simulink model "Servo_PID"  (R2013b)
settings: Solver=ode5  SolverMode=SingleTasking  StartTime=0.0  StopTime=30  FixedStep=0.002  RelTol=1e-3  AbsTol=1e-6
undefined symbols (not defined in the file): a, b, ksi, ksie, lambda, omega, omegae, RTDAC4PCIBaseAddress, Tfiltra, Tsampling
settings Model: SimulationMode=external  ExtModeTrigDuration=20000  ExtModeTrigLevel=0.400000  Creator=jims  LastModifiedBy=Admin
settings DataIOCC: ExternalInput=[]  InitialState=[]  LimitDataPoints=off  MaxDataPoints=5000  SignalLoggingSaveFormat=ModelDataLogs  SaveOutput=off  SaveTime=off  SignalLoggingName=sigsOut
settings OptimizationCC: BooleanDataType=off  ExpressionDepthLimit=2147483647  InitFltsAndDblsToZero=on
settings DebuggingCC: SaveWithParameterizedLinksMsg=none  SignalResolutionControl=TryResolveAllWithWarning  SolverPrmCheckMsg=none  MultiTaskDSMMsg=warning  MultiTaskCondExecSysMsg=none  IntegerOverflowMsg=none  FcnCallInpInsideContextMsg=UseLocalSettings  StateNameClashWarn=warning
settings HardwareCC: ProdIntDivRoundTo=Zero  ProdEndianess=LittleEndian  ProdHWDeviceType=Generic->32-bit x86 compatible
settings RTWCC: SystemTargetFile=rtwin.tlc  TemplateMakefile=rtwin.tmf  Description=Real-Time Windows Target  ProcessScript=rtwin_make_rtw_hook  IncludeERTFirstTime=on  RTWCompilerOptimization=On
settings CodeAppCC: MaxIdLength=95
settings RTWinTargetCC: TargetLibSuffix=_rtwin.lib  TargetPreCompLibLocation=C:\Program Files\MATLAB\R2013b\toolbox\rtw\targets\rtwin\lib\win64  CodeReplacementLibrary=ANSI_C  RTWinDir=C:/PROGRA~1/MATLAB/R2013b/toolbox/rtw/targets/rtwin  TargetArch=win64

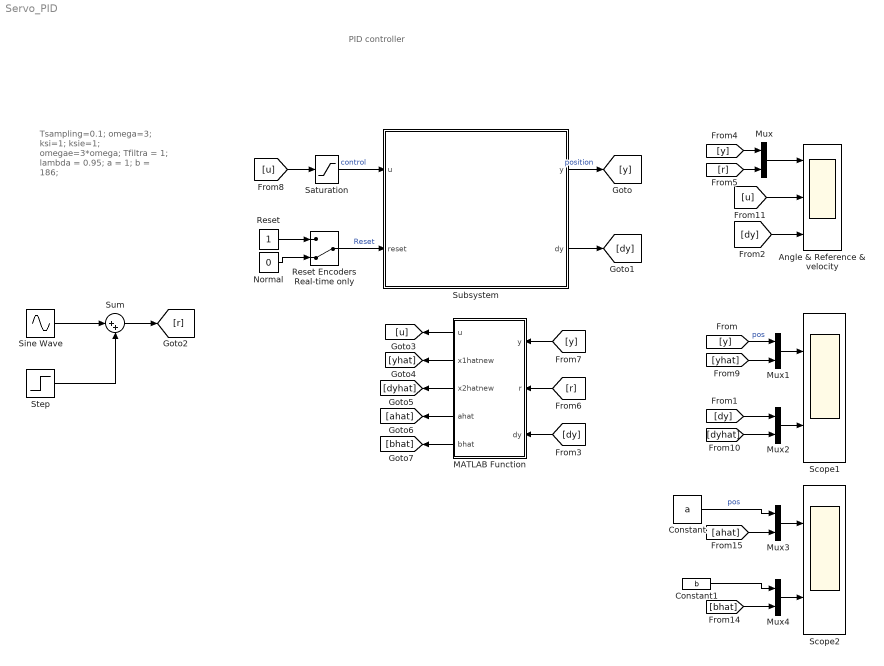
== system Servo_PID ==
  note: Tsampling=0.1;
      | omega=3;
      | ksi=1;
      | ksie=1;
      | omegae=3*omega;
      | Tfiltra = 1;
      | lambda = 0.95;
      | a = 1;
      | b = 186;
  note: PID controller
  Angle & Reference & velocity : Scope  NumInputPorts=3
      settings: ShowLegends=on  TimeRange=30  YMin=250~-0.175~-16  YMax=350~0.075~7  SaveName=PD_C  MaxDataPoints=20000  Decimation=10
  Constant : Constant  Value=a
  Constant1 : Constant  Value=b
  MATLAB Function : MATLAB Function  TreatAsAtomicUnit=on
  Mux{,1..4} (5 alike) : Mux  Inputs=2
  Normal : Constant  Value=0
  Reset : Constant
  Reset Encoders Real-time only : ManualSwitch  CurrentSetting=0
  Saturation : Saturate  UpperLimit=1  LowerLimit=-1
  Scope1 : Scope  NumInputPorts=2
      settings: ShowLegends=on  YMin=275~0  YMax=350~19
  Scope2 : Scope  NumInputPorts=2
      settings: ShowLegends=on  YMin=275~0  YMax=350~19
  Sine Wave : Sin  Amplitude=50  Frequency=2*pi/20  SampleTime=0
  Step : Step  After=300  SampleTime=0
  Subsystem : Subsystem
  Sum : Sum  Inputs=|++
  wires:
  Normal/1 -> Reset Encoders Real-time only/2
  Reset/1 -> Reset Encoders Real-time only/1
  Saturation/1 -> Subsystem/1(u)  "control"
  Reset Encoders Real-time only/1 -> Subsystem/2(reset)  "Reset"
  Mux/1 -> Angle & Reference & velocity/1
  Subsystem/2(dy) -> [dy]
  Subsystem/1(y) -> [y]  "position"
  [dy] -> Angle & Reference & velocity/3
  [dy] -> MATLAB Function/3(dy)
  [y] -> Mux/1
  Sine Wave/1 -> Sum/1
  Step/1 -> Sum/2
  Sum/1 -> [r]
  [r] -> Mux/2
  [r] -> MATLAB Function/2(r)
  [y] -> MATLAB Function/1(y)
  MATLAB Function/1(u) -> [u]
  [u] -> Saturation/1
  Mux1/1 -> Scope1/1
  Mux2/1 -> Scope1/2
  [y] -> Mux1/1  "pos"
  [dy] -> Mux2/1
  MATLAB Function/2(x1hatnew) -> [yhat]
  MATLAB Function/3(x2hatnew) -> [dyhat]
  [yhat] -> Mux1/2
  [dyhat] -> Mux2/2
  [u] -> Angle & Reference & velocity/2
  MATLAB Function/4(ahat) -> [ahat]
  MATLAB Function/5(bhat) -> [bhat]
  Mux3/1 -> Scope2/1
  Mux4/1 -> Scope2/2
  Constant/1 -> Mux3/1  "pos"
  Constant1/1 -> Mux4/1
  [ahat] -> Mux3/2
  [bhat] -> Mux4/2

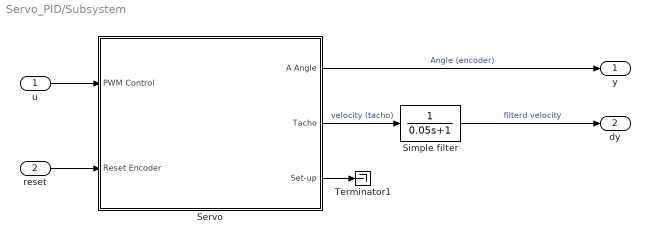
== system Servo_PID/Subsystem ==
  u : Inport
  reset : Inport  Port=2
  Servo : Subsystem  mask{BaseAddress=RTDAC4PCIBaseAddress(-1,-1), T0=0.002}
      mask prompts: BaseAddress "Base Address:"; T0 "Sampling Period:"
      mask Display: image(imread('Servo.JPG'))
  Simple filter : TransferFcn  Denominator=[0.05 1]
  Terminator1 : Terminator
  y : Outport
  dy : Outport  Port=2
  wires:
  Simple filter/1 -> dy/1  "filterd velocity"
  Servo/1(A Angle) -> y/1  "Angle (encoder)"
  reset/1 -> Servo/2(Reset Encoder)
  Servo/2(Tacho) -> Simple filter/1  "velocity (tacho)"
  Servo/3(Set-up) -> Terminator1/1
  u/1 -> Servo/1(PWM Control)

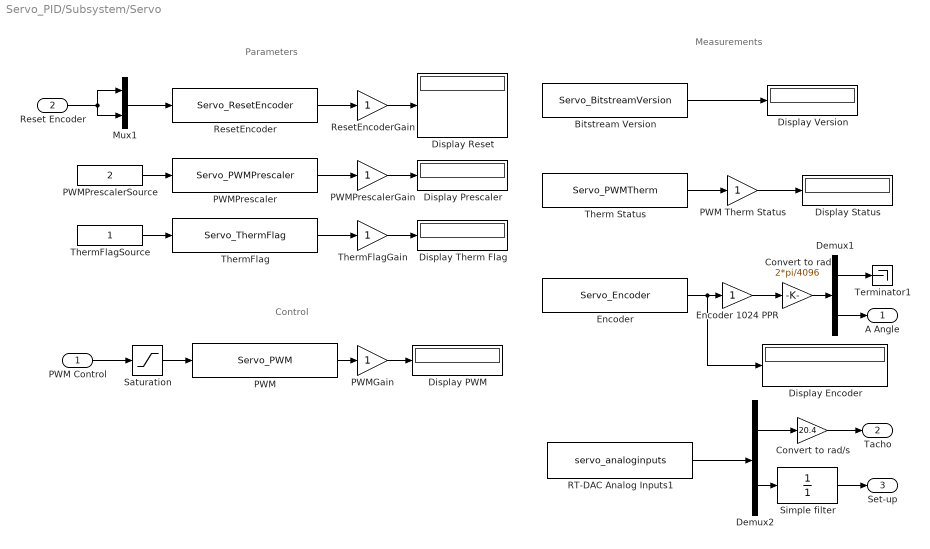
== system Servo_PID/Subsystem/Servo ==
  note: Parameters
  note: Control
  note: Measurements
  PWM Control : Inport
  Reset Encoder : Inport  Port=2
  Bitstream Version : S-Function  FunctionName=Servo_BitstreamVersion  Parameters=BaseAddress, T0  EnableBusSupport=off
  Convert to rad : Gain  Gain=2*pi/4096  SaturateOnIntegerOverflow=on  OutDataTypeStr=Inherit: Same as input  ParamDataTypeStr=Inherit: Same as input
  Convert to rad/s : Gain  Gain=20.4  SaturateOnIntegerOverflow=on  OutDataTypeStr=Inherit: Same as input  ParamDataTypeStr=Inherit: Same as input
  Demux1 : Demux  Outputs=2
  Demux2 : Demux  Outputs=2
  Display Encoder : Display
  Display PWM : Display
  Display Prescaler : Display
  Display Reset : Display
  Display Status : Display
  Display Therm Flag : Display
  Display Version : Display
  Encoder : S-Function  FunctionName=Servo_Encoder  Parameters=BaseAddress, T0  EnableBusSupport=off
  Encoder 1024 PPR : Gain  SaturateOnIntegerOverflow=on  OutDataTypeStr=Inherit: Same as input  ParamDataTypeStr=Inherit: Same as input
  Mux1 : Mux  Inputs=2
  PWM : S-Function  FunctionName=Servo_PWM  Parameters=BaseAddress, T0  EnableBusSupport=off
  PWM Therm Status : Gain  SaturateOnIntegerOverflow=on  OutDataTypeStr=Inherit: Same as input  ParamDataTypeStr=Inherit: Same as input
  PWMGain : Gain  SaturateOnIntegerOverflow=on  OutDataTypeStr=Inherit: Same as input  ParamDataTypeStr=Inherit: Same as input
  PWMPrescaler : S-Function  FunctionName=Servo_PWMPrescaler  Parameters=BaseAddress, T0  EnableBusSupport=off
  PWMPrescalerGain : Gain  SaturateOnIntegerOverflow=on  OutDataTypeStr=Inherit: Same as input  ParamDataTypeStr=Inherit: Same as input
  PWMPrescalerSource : Constant  Value=2
  RT-DAC Analog Inputs1 : S-Function  FunctionName=servo_analoginputs  Parameters=BaseAddress, [1 0], [1 1], T0  EnableBusSupport=off
  ResetEncoder : S-Function  FunctionName=Servo_ResetEncoder  Parameters=BaseAddress, T0  EnableBusSupport=off
  ResetEncoderGain : Gain  SaturateOnIntegerOverflow=on  OutDataTypeStr=Inherit: Same as input  ParamDataTypeStr=Inherit: Same as input
  Saturation : Saturate  UpperLimit=1  LowerLimit=-1
  Simple filter : TransferFcn  Denominator=[0.0 1]
  Terminator1 : Terminator
  Therm Status : S-Function  FunctionName=Servo_PWMTherm  Parameters=BaseAddress, T0  EnableBusSupport=off
  "ThermFlag " : S-Function  FunctionName=Servo_ThermFlag  Parameters=BaseAddress, T0  EnableBusSupport=off
  ThermFlagGain : Gain  SaturateOnIntegerOverflow=on  OutDataTypeStr=Inherit: Same as input  ParamDataTypeStr=Inherit: Same as input
  ThermFlagSource : Constant
  A Angle : Outport
  Tacho : Outport  Port=2
  Set-up : Outport  Port=3
  wires:
  Encoder 1024 PPR/1 -> Convert to rad/1
  Encoder/1 -> Encoder 1024 PPR/1, Display Encoder/1
  Saturation/1 -> PWM/1
  PWM/1 -> PWMGain/1
  PWMGain/1 -> Display PWM/1
  ResetEncoder/1 -> ResetEncoderGain/1
  PWMPrescaler/1 -> PWMPrescalerGain/1
  Mux1/1 -> ResetEncoder/1
  PWMPrescalerSource/1 -> PWMPrescaler/1
  ResetEncoderGain/1 -> Display Reset/1
  PWMPrescalerGain/1 -> Display Prescaler/1
  PWM Control/1 -> Saturation/1
  Convert to rad/1 -> Demux1/1
  Therm Status/1 -> PWM Therm Status/1
  PWM Therm Status/1 -> Display Status/1
  Bitstream Version/1 -> Display Version/1
  Reset Encoder/1 -> Mux1/1, Mux1/2
  "ThermFlag "/1 -> ThermFlagGain/1
  ThermFlagSource/1 -> "ThermFlag "/1
  ThermFlagGain/1 -> Display Therm Flag/1
  Demux1/1 -> Terminator1/1
  Demux1/2 -> A Angle/1
  RT-DAC Analog Inputs1/1 -> Demux2/1
  Demux2/2 -> Simple filter/1
  Demux2/1 -> Convert to rad/s/1
  Convert to rad/s/1 -> Tacho/1
  Simple filter/1 -> Set-up/1

== matlab function Servo_PID/MATLAB Function ==
  settings: updateMethod=DISCRETE  sampleTime=Tsampling
  data: u output; y input; r input; Tsampling parameter; omega parameter; ksi parameter; dy input; omegae parameter; ksie parameter; x1hatnew output; x2hatnew output; Tfiltra parameter; lambda parameter; ahat output; bhat output
function [u, x1hatnew, x2hatnew, ahat, bhat] = fcn(y, r, Tsampling, omega, ksi, dy, omegae, ksie, Tfiltra, lambda)

persistent x1hat x2hat uprev
if isempty(x1hat) || isempty(x2hat) || isempty(uprev)
    x1hat=0;
    x2hat=0;
    uprev = 0;
end

persistent ufp x2fp
if isempty(ufp)
    ufp = 0;
    x2fp = 0;
end

% Filtering
p = exp(-Tsampling/Tfiltra);

uf = p * ufp + (1-p) * uprev;
ufp = uf;

x2f = p * x2fp + (1-p) * dy;
dx2f = (x2f - x2fp)/Tsampling;
x2fp = x2f;

% Kalman
persistent P theta
if isempty(P)
    P = 50*eye(2);
    theta = [0 0]';
end

phi = [-x2f uf]';
z = dx2f;
P = (1/lambda) * (P + (P'*(phi*phi')*P)/(lambda + phi'*P*phi));
theta = theta + P*phi*(z-phi'*theta);
ahat = theta(1);
bhat = theta(2);


% Control & observer
a=1;
b=186;

k1=omega^2/b;
k2=(2*ksi*omega-a)/b;
kr=k1;

L1=2*ksie*omegae-a;
L2=omegae^2-a*L1;

x1hatnew=x1hat+Tsampling*(x2hat+L1*(y-x1hat));
x2hatnew=x2hat+Tsampling*(-a*x2hat+b*uprev+L2*(y-x1hat));
x1hat=x1hatnew;
x2hat=x2hatnew;

% u=-k1*y-k2*dy+kr*r;
u=-k1*x1hat-k2*x2hat+kr*r;

if u>1
    u = 1;
elseif u<-1
    u = -1;
end;

uprev = u;
